simulink model "sol1"  (R2018a)
settings: Solver=VariableStepAuto  StartTime=0.0  StopTime=30.0  RelTol=1e-3
settings Model: Creator=soutrik  LastModifiedBy=soutrik

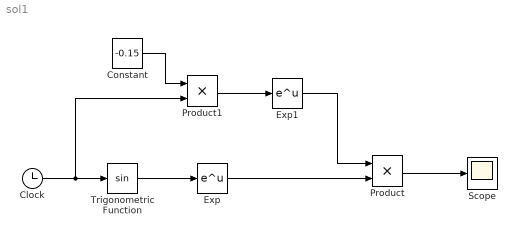
== system sol1 ==
  Clock : Clock
  Constant : Constant  Value=-0.15
  Exp : Math  SaturateOnIntegerOverflow=on
  Exp1 : Math  SaturateOnIntegerOverflow=on
  Product : Product
  Product1 : Product
  Scope : Scope
  Trigonometric Function : Trigonometry
  wires:
  Trigonometric Function/1 -> Exp/1
  Clock/1 -> Product1/2, Trigonometric Function/1
  Exp/1 -> Product/2
  Constant/1 -> Product1/1
  Product1/1 -> Exp1/1
  Exp1/1 -> Product/1
  Product/1 -> Scope/1
